simulink model "LCK"  (R2018b)
settings: Solver=FixedStepDiscrete  StartTime=0.0  StopTime=inf  FixedStep=0.01  RelTol=1e-3
PostLoadFcn:
  | if any(exist('dsrtsu_mdlpostloadfcn', 'file') ~= 0), dsrtsu_mdlpostloadfcn('Execute', bdroot); end
values from neighbouring files (symbols this model uses):
  C_DEG2RAD = 0.0175    [LCK_Macro.sldd]
  C_KPH2MPS = 0.2778    [LCK_Macro.sldd]
  C_NEARZERO = 0.0001    [LCK_Macro.sldd]
  C_ONE = 1.0    [LCK_Macro.sldd]
  C_RAD2DEG = 57.2958    [LCK_Macro.sldd]
  C_ZERO = 0.0    [LCK_Macro.sldd]
  k_accel_pedal_pos_per_speed_x : value not decoded    [LCK_LogicPara.sldd]
  k_accel_pedal_pos_per_speed_z : value not decoded    [LCK_LogicPara.sldd]
  k_brake_suprress_hold = 1000.0    [LCK_LogicPara.sldd]
  k_driver_appl_torque_filt = 50.0    [LCK_LogicPara.sldd]
  k_driver_suppression_hold_time = 3000.0    [LCK_LogicPara.sldd]
  k_hands_on_wheel_hold_msec = 500.0    [LCK_LogicPara.sldd]
  k_hands_on_wheel_torque_hi = 0.2    [LCK_LogicPara.sldd]
  k_hands_on_wheel_torque_lo = 0.15    [LCK_LogicPara.sldd]
  k_handsoff_delay_cycles = 50.0    [LCK_LogicPara.sldd]
  k_handsoff_torq_Lo_CR = 0.3    [LCK_LogicPara.sldd]
  k_handson_delay_cycles = 5.0    [LCK_LogicPara.sldd]
  k_HighAccel_suppress_hold = 3000.0    [LCK_LogicPara.sldd]
  k_HLR_suprress_hold = 3000.0    [LCK_LogicPara.sldd]
  k_hs_StrAng_CR_threshold_z : value not decoded    [LCK_LogicPara.sldd]
  k_LC_Exit_Switch = 0.0    [LCK_LogicPara.sldd]
  k_LCG_Configured = 1.0    [LCK_LogicPara.sldd]
  k_LCK_A0_Rdy2Act_UseConst = 0.0    [LCK_LogicPara.sldd]
  k_LCK_A0Fac_ActSta : value not decoded    [LCK_CtrlPara.sldd]
  k_LCK_A0Fac_DrvStm : value not decoded    [LCK_CtrlPara.sldd]
  k_LCK_A0Shift_LftCurv : value not decoded    [LCK_CtrlPara.sldd]
  k_LCK_A0Shift_RgtCurv : value not decoded    [LCK_CtrlPara.sldd]
  k_LCK_A0Shift_StraLan = 0.0    [LCK_CtrlPara.sldd]
  k_LCK_A0ShiftFac_Dy_LftCurv : value not decoded    [LCK_CtrlPara.sldd]
  k_LCK_A0ShiftFac_Dy_RgtCurv : value not decoded    [LCK_CtrlPara.sldd]
  k_LCK_A0ShiftFac_Vspd : value not decoded    [LCK_CtrlPara.sldd]
  k_LCK_accel_inhibit_thold = 35.0    [LCK_LogicPara.sldd]
  k_LCK_Active2Ready_Mask = 255.0    [LCK_LogicPara.sldd]
  k_LCK_CvatRateBks : value not decoded    [LCK_CtrlPara.sldd]
  k_LCK_CvatrBks : value not decoded    [LCK_CtrlPara.sldd]
  k_LCK_DFac_Dy : value not decoded    [LCK_CtrlPara.sldd]
  k_LCK_DFac_Dy_Curv : value not decoded    [LCK_CtrlPara.sldd]
  k_LCK_DFac_HaCurCen : value not decoded    [LCK_CtrlPara.sldd]
  k_LCK_DFac_HaCurSid : value not decoded    [LCK_CtrlPara.sldd]
  k_LCK_DFac_HadCurCen : value not decoded    [LCK_CtrlPara.sldd]
  k_LCK_DFac_HadCurSid : value not decoded    [LCK_CtrlPara.sldd]
  k_LCK_DFac_HadStrCen : value not decoded    [LCK_CtrlPara.sldd]
  k_LCK_DFac_HadStrSid : value not decoded    [LCK_CtrlPara.sldd]
  k_LCK_DFac_HaStrCen : value not decoded    [LCK_CtrlPara.sldd]
  k_LCK_DFac_HaStrSid : value not decoded    [LCK_CtrlPara.sldd]
  k_LCK_DFac_Rad : value not decoded    [LCK_CtrlPara.sldd]
  k_LCK_DFac_SA_CurCen : value not decoded    [LCK_CtrlPara.sldd]
  k_LCK_DFac_SA_CurSid : value not decoded    [LCK_CtrlPara.sldd]
  k_LCK_DFac_SA_StrCen : value not decoded    [LCK_CtrlPara.sldd]
  k_LCK_DFac_SA_StrSid : value not decoded    [LCK_CtrlPara.sldd]
  k_LCK_DFac_SS_CurCen : value not decoded    [LCK_CtrlPara.sldd]
  k_LCK_DFac_SS_CurSid : value not decoded    [LCK_CtrlPara.sldd]
  k_LCK_DFac_SS_StrCen : value not decoded    [LCK_CtrlPara.sldd]
  k_LCK_DFac_SS_StrSid : value not decoded    [LCK_CtrlPara.sldd]
  k_LCK_DFac_Vspd : value not decoded    [LCK_CtrlPara.sldd]
  k_LCK_DlyTm_DrvStim = 0.2    [LCK_CtrlPara.sldd]
  k_LCK_DTermMax = 2.0    [LCK_CtrlPara.sldd]
  k_LCK_DyBks_Curv : value not decoded    [LCK_CtrlPara.sldd]
  k_LCK_Enable_POOnly = 1.0    [LCK_LogicPara.sldd]
  k_LCK_Entry_DistBuffer = 0.1    [LCK_LogicPara.sldd]
  k_LCK_Fac_Vspd2RngThr_FalRec = 0.23    [LCK_CtrlPara.sldd]
  k_LCK_Ffw_CvatSwh = 0.0    [LCK_CtrlPara.sldd]
  k_LCK_Ffw_DyBks : value not decoded    [LCK_CtrlPara.sldd]
  k_LCK_Ffw_TimCon_CmdFlt = 0.0    [LCK_CtrlPara.sldd]
  k_LCK_FfwDeltaFac_Rad_Lft : value not decoded    [LCK_CtrlPara.sldd]
  k_LCK_FfwDeltaFac_Rad_Rgt : value not decoded    [LCK_CtrlPara.sldd]
  k_LCK_FfwDeltaFac_Vspd : value not decoded    [LCK_CtrlPara.sldd]
  k_LCK_FfwFac_CvatRate_Lft : value not decoded    [LCK_CtrlPara.sldd]
  k_LCK_FfwFac_CvatRate_Rgt : value not decoded    [LCK_CtrlPara.sldd]
  k_LCK_FfwFac_Dy : value not decoded    [LCK_CtrlPara.sldd]
  k_LCK_FfwFac_Rad_Lft : value not decoded    [LCK_CtrlPara.sldd]
  k_LCK_FfwFac_Rad_Rgt : value not decoded    [LCK_CtrlPara.sldd]
  k_LCK_FfwFac_Vspd : value not decoded    [LCK_CtrlPara.sldd]
  k_LCK_FfwTorq_Cvat : value not decoded    [LCK_CtrlPara.sldd]
  k_LCK_HAFac_ActSta : value not decoded    [LCK_CtrlPara.sldd]
  k_LCK_HAFac_DrvStm : value not decoded    [LCK_CtrlPara.sldd]
  k_LCK_HaloTime = 2000.0    [LCK_LogicPara.sldd]
  k_LCK_HaloTime_Switch = 0.0    [LCK_LogicPara.sldd]
  k_LCK_HARFac_ActSta : value not decoded    [LCK_CtrlPara.sldd]
  k_LCK_HARFac_DrvStm : value not decoded    [LCK_CtrlPara.sldd]
  k_LCK_Hed_DyBks : value not decoded    [LCK_CtrlPara.sldd]
  k_LCK_HedAngDiffX : value not decoded    [LCK_CtrlPara.sldd]
  k_LCK_HedAngRateDiffX : value not decoded    [LCK_CtrlPara.sldd]
  k_LCK_HndsOnWhel_DlyTm_Idl2Rdy = 0.0    [LCK_LogicPara.sldd]
  k_LCK_host_veh_width = 1.86    [LCK_LogicPara.sldd]
  k_LCK_Idle2Ready_Mask = 239.0    [LCK_LogicPara.sldd]
  k_LCK_Junc_SusTime = 1.0    [LCK_LogicPara.sldd]
  k_LCK_KpKdDecSlopeLmt = 10.0    [LCK_CtrlPara.sldd]
  k_LCK_KpKdIncSlopeLmt = 5.0    [LCK_CtrlPara.sldd]
  k_LCK_Lat_Ctrl_DFac_Lft = 1.0    [LCK_CtrlPara.sldd]
  k_LCK_Lat_Ctrl_DFac_Rgt = 1.05    [LCK_CtrlPara.sldd]
  k_LCK_Lat_Ctrl_Kd = 0.8    [LCK_CtrlPara.sldd]
  k_LCK_Lat_Ctrl_Ki = 0.5    [LCK_CtrlPara.sldd]
  k_LCK_Lat_Ctrl_Kp = 0.7    [LCK_CtrlPara.sldd]
  k_LCK_Lat_Ctrl_Kp_NearGain = 0.7    [LCK_CtrlPara.sldd]
  k_LCK_Lat_Ctrl_PFac_Lft = 1.0    [LCK_CtrlPara.sldd]
  k_LCK_Lat_Ctrl_PFac_Rgt = 1.05    [LCK_CtrlPara.sldd]
  k_LCK_Lat_Ctrl_TimCon_CmdFlt = 5.0    [LCK_CtrlPara.sldd]
  k_LCK_Lat_DFac_Rad : value not decoded    [LCK_CtrlPara.sldd]
  k_LCK_Lat_DFac_SS_Cur : value not decoded    [LCK_CtrlPara.sldd]
  k_LCK_Lat_DFac_SS_Str : value not decoded    [LCK_CtrlPara.sldd]
  k_LCK_Lat_DFac_Vspd : value not decoded    [LCK_CtrlPara.sldd]
  k_LCK_Lat_DyBks : value not decoded    [LCK_CtrlPara.sldd]
  k_LCK_Lat_IFac_Rad : value not decoded    [LCK_CtrlPara.sldd]
  k_LCK_Lat_IFac_Vspd : value not decoded    [LCK_CtrlPara.sldd]
  k_LCK_Lat_ILmtFac_Dy_CurvLan : value not decoded    [LCK_CtrlPara.sldd]
  k_LCK_Lat_ILmtFac_Dy_StraLan : value not decoded    [LCK_CtrlPara.sldd]
  k_LCK_Lat_ILmtFac_Rad : value not decoded    [LCK_CtrlPara.sldd]
  k_LCK_Lat_ILmtFac_Rad_NearGain = 1.0    [LCK_CtrlPara.sldd]
  k_LCK_Lat_ILmtFac_Vspd_CurvLan : value not decoded    [LCK_CtrlPara.sldd]
  k_LCK_Lat_ILmtFac_Vspd_StraLan : value not decoded    [LCK_CtrlPara.sldd]
  k_LCK_Lat_ITermLmt_Dy = 1.0    [LCK_CtrlPara.sldd]
  k_LCK_Lat_KpKdDecSlopeLmt = 10.0    [LCK_CtrlPara.sldd]
  k_LCK_Lat_KpKdIncSlopeLmt = 10.0    [LCK_CtrlPara.sldd]
  k_LCK_Lat_PFac_Dy_InnLftCur : value not decoded    [LCK_CtrlPara.sldd]
  k_LCK_Lat_PFac_Dy_InnRgtCur : value not decoded    [LCK_CtrlPara.sldd]
  k_LCK_Lat_PFac_Dy_OutLftCur : value not decoded    [LCK_CtrlPara.sldd]
  k_LCK_Lat_PFac_Dy_OutRgtCur : value not decoded    [LCK_CtrlPara.sldd]
  k_LCK_Lat_PFac_Dy_Str : value not decoded    [LCK_CtrlPara.sldd]
  k_LCK_Lat_PFac_Rad : value not decoded    [LCK_CtrlPara.sldd]
  ... (+153 more)
undefined symbols (not defined in the file or in its folder): k_LCK_CurvBks, K_LCK_SPA0A1A2_LMRngCmp_y
libraries: LateralControl_fcns_lib x59, simulink x24
(part 30 of 47)

== system LCK/Lateral_Control_Module/LCK_State_Ctrl/LCK_Mode_Transition/Determination_of_Junction ==
  SP_max_range : Inport
  VIS_LANE_LEFT_INDIVID_RANGE : Inport  Port=2
  VIS_LANE_RIGHT_INDIVID_RANGE : Inport  Port=3
  SP_type : Inport  Port=4
  Constant14 : Constant  Tag={'output',{'name','$P','class','EXTERN_MACRO','type','UInt8'},'date',737531.64011871524}  Description=_GACA26P4.LCK.000_9_  Value=TJA_SP_TYPE_BLMONLY
  Constant17 : Constant  Tag={'output',{'name','$P','class','EXTERN_MACRO','type','UInt8'},'date',737531.6327261111}  Description=_GACA26P4.LCK.000_10_  Value=TJA_SP_TYPE_BLMONLY
  Data Type Conversion88 : DataTypeConversion  Description=_GACA26P4.LCK.000_13_
  Data Type Conversion89 : DataTypeConversion  Description=_GACA26P4.LCK.000_14_
  Delay_Trig : LateralControl_fcns_lib/Delay_Trig  SystemSampleTime=-1
  Logical Operator155 : Logic  Tag={'date',737531.60590739583}  Description=_GACA26P4.LCK.000_31_  Operator=NOT  AllPortsSameDT=off  OutDataTypeStr=boolean
  Logical Operator157 : Logic  Tag={'date',737531.60590834497}  Description=_GACA26P4.LCK.000_32_  Inputs=3  AllPortsSameDT=off  OutDataTypeStr=boolean
  MinMax3 : MinMax  Tag={'output',{'type','Float32'},'date',737531.79517509264}  Description=_GACA26P4.LCK.000_35_  Inputs=2  OutDataTypeStr=single
  Relational Operator204 : RelationalOperator  Tag={'date',737531.60601302085}  Description=_GACA26P4.LCK.000_37_  Operator===  OutDataTypeStr=boolean  RndMeth=Nearest
  Relational Operator205 : RelationalOperator  Tag={'date',737531.60601353005}  Description=_GACA26P4.LCK.000_38_  Operator=<  OutDataTypeStr=boolean  RndMeth=Nearest
  Relational Operator207 : RelationalOperator  Tag={'date',737531.60601446754}  Description=_GACA26P4.LCK.000_39_  Operator===  OutDataTypeStr=boolean  RndMeth=Nearest
  Relational Operator208 : RelationalOperator  Tag={'date',737531.60601498839}  Description=_GACA26P4.LCK.000_40_  Operator=<  OutDataTypeStr=boolean  RndMeth=Nearest
  Relational Operator209 : RelationalOperator  Tag={'date',737531.60601548606}  Description=_GACA26P4.LCK.000_41_  Operator===  OutDataTypeStr=boolean  RndMeth=Nearest
  Signal_Sustain_With_Clear : LateralControl_fcns_lib/Signal_Sustain_With_Clear  Description=_GWMAB30P4.Latctrl.000_162_  SystemSampleTime=-1
  Switch67 : Switch  Tag={'output',{'type','Float32'},'threshold',{'type','Int32'},'date',737531.80936515052}  Description=_GACA26P4.LCK.000_47_  Threshold=0.5
  Switch69 : Switch  Tag={'output',{'type','Float32'},'threshold',{'type','Int32'},'date',737531.80957618053}  Description=_GACA26P4.LCK.000_49_  Threshold=0.5
  Unit Delay11 : UnitDelay  Tag={'output',{'inheritscaling',1},'state',{'type','Int32'},'date',737531.81173646986}  Description=_GACA26P4.LCK.000_54_  SampleTime=-1
  Unit Delay6 : UnitDelay  Tag={'output',{'inheritscaling',1},'state',{'type','Int32'},'date',737531.80972199072}  Description=_GACA26P4.LCK.000_55_  SampleTime=-1
  Unit Delay7 : UnitDelay  Tag={'output',{'inheritscaling',1},'state',{'type','Int32'},'date',737531.80965883099}  Description=_GACA26P4.LCK.000_56_  SampleTime=-1
  k_LCK_Junc_SusTime : Constant  Tag={'output',{'name','$P','class','EXTERN_CAL','type','Float32'},'date',737531.6374285185}  Description=_GACA26P4.LCK.000_59_  Value=k_LCK_Junc_SusTime
  k_LCK_MinJunction_Range : Constant  Tag={'output',{'name','$P','class','EXTERN_CAL','type','Float32'},'date',737531.63752556709}  Description=_GACA26P4.LCK.000_60_  Value=k_LCK_MinJunction_Range
  k_LCK_Range_Drop_MinDur : Constant  Tag={'output',{'name','$P','class','EXTERN_CAL','type','Float32'},'date',737531.63768747682}  Description=_GACA26P4.LCK.000_62_  Value=k_LCK_Range_Drop_MinDur
  k_LCK_UseSP_MaxRange : Constant  Tag={'output',{'name','$P','class','EXTERN_CAL','type','Bool'},'date',737531.64552409726}  Description=_GACA26P4.LCK.000_71_  Value=k_LCK_UseSP_MaxRange  VectorParams1D=off
  Junction : Outport
  wires:
  Relational Operator208/1 -> Logical Operator157/2
  Unit Delay6/1 -> Switch69/1
  Switch67/1 -> [LM_Range], Unit Delay7/1, Relational Operator209/1, Unit Delay11/1
  Switch69/1 -> Relational Operator205/2, Unit Delay6/1
  Relational Operator207/1 -> Logical Operator155/1
  Constant17/1 -> Relational Operator207/1
  [LM_Range] -> Relational Operator208/1
  Relational Operator205/1 -> Data Type Conversion89/1
  k_LCK_MinJunction_Range/1 -> Relational Operator208/2
  MinMax3/1 -> Switch67/3
  Logical Operator155/1 -> Data Type Conversion88/1
  k_LCK_Junc_SusTime/1 -> Signal_Sustain_With_Clear/2
  Delay_Trig/1 -> Signal_Sustain_With_Clear/1
  Constant14/1 -> Relational Operator204/1
  VIS_LANE_LEFT_INDIVID_RANGE/1 -> MinMax3/1
  Unit Delay11/1 -> Relational Operator209/2
  Signal_Sustain_With_Clear/1 -> Logical Operator157/3
  Logical Operator157/1 -> Junction/1
  Relational Operator204/1 -> Logical Operator157/1
  Data Type Conversion88/1 -> Signal_Sustain_With_Clear/3
  [SP_type] -> Relational Operator204/2
  Unit Delay7/1 -> Switch69/3
  [LM_Range] -> Relational Operator205/1
  Relational Operator209/1 -> Switch69/2
  k_LCK_UseSP_MaxRange/1 -> Switch67/2
  k_LCK_Range_Drop_MinDur/1 -> Delay_Trig/2
  Data Type Conversion89/1 -> Delay_Trig/1
  SP_type/1 -> [SP_type], Relational Operator207/2
  SP_max_range/1 -> Switch67/1
  VIS_LANE_RIGHT_INDIVID_RANGE/1 -> MinMax3/2

== system LCK/Lateral_Control_Module/LCK_State_Ctrl/LCK_Mode_Transition/Determination_of_Lat_Ctrl_Req ==
  LCK_Switch : Inport
  TJA_LatCtrl_Rq_Input : Inport  Port=2
  veh_speed_kph : Inport  Port=3
  Constant1 : Constant  Value=k_LCK_TJALCK_SWSpeed
  Constant20 : Constant  Tag={'output',{'type','Int32'},'date',737184.60397293977}  Description=_GWMAB30P2.LCK.000_1071_
  LCK_TJA_LatRq_Manager : Stateflow chart  TreatAsAtomicUnit=on
  Switch6 : Switch  Tag={'output',{'inheritscaling',1},'threshold',{'type','Int32','scalar',1},'date',737243.50339983799}  Description=_GWMAB30P2.LCK.000_1196_  Threshold=0.5
  k_LCK_VisionOnly : Constant  Tag={'output',{'name','$P','class','EXTERN_CAL','type','Bool'},'date',737246.86429052078}  Description=_GWMAB30P2.LCK.000_1268_  Value=k_LCK_VisionOnly
  LCKON_TJAOFF : Outport
  TJA_LatCtrl_Rq : Outport  Port=2
  wires:
  veh_speed_kph/1 -> LCK_TJA_LatRq_Manager/3(VehicleSpd)
  Constant20/1 -> Switch6/1
  k_LCK_VisionOnly/1 -> Switch6/2
  Switch6/1 -> TJA_LatCtrl_Rq/1
  Constant1/1 -> LCK_TJA_LatRq_Manager/4(k_LCK_TJALCK_SWSpeed)
  LCK_TJA_LatRq_Manager/2(LatRq) -> Switch6/3
  TJA_LatCtrl_Rq_Input/1 -> LCK_TJA_LatRq_Manager/1(TJA_LatCtrl_Rq)
  LCK_TJA_LatRq_Manager/1(LCKON_TJAOFF) -> LCKON_TJAOFF/1
  LCK_Switch/1 -> LCK_TJA_LatRq_Manager/2(LCK_Switch)

== system LCK/Lateral_Control_Module/LCK_State_Ctrl/LCK_Mode_Transition/Determination_of_OFF2IDLE ==
  TJA_Switch : Inport
  LCK_Switch : Inport  Port=2
  Logical Operator : Logic  Tag={'date',737184.60397559032}  Description=_GWMAB30P2.LCK.000_1090_  Operator=OR  AllPortsSameDT=off  OutDataTypeStr=boolean
  OFF2IDLE : Outport
  wires:
  TJA_Switch/1 -> Logical Operator/1
  LCK_Switch/1 -> Logical Operator/2
  Logical Operator/1 -> OFF2IDLE/1

== system LCK/Lateral_Control_Module/LCK_State_Ctrl/LCK_Mode_Transition/Determination_of_OFF2READY ==
  TJA_Switch : Inport
  LCK_Switch : Inport  Port=2
  IDLE2READY : Inport  Port=3
  Logical Operator48 : Logic  Tag={'date',737237.63746775466}  Description=_GWMAB30P3.LCK.000_66_  Operator=OR  AllPortsSameDT=off  OutDataTypeStr=boolean
  Logical Operator49 : Logic  Tag={'date',737237.63746789354}  Description=_GWMAB30P3.LCK.000_67_  Inputs=3  AllPortsSameDT=off  OutDataTypeStr=boolean
  Relational_Operator6 : RelationalOperator  Tag={'date',737237.63747481478}  Description=_GWMAB30P3.LCK.000_109_  Operator===  OutDataTypeStr=boolean  RndMeth=Nearest
  ZERO7 : Constant  Tag={'output',{'type','Int32'},'date',737296.79743047454}  Description=_GWMAB30P3.LCK.000_124_  Value=0  SampleTime=-1
  OFF2READY : Outport
  wires:
  IDLE2READY/1 -> Logical Operator49/2
  Logical Operator48/1 -> Logical Operator49/1
  TJA_Switch/1 -> Logical Operator48/1
  ZERO7/1 -> Relational_Operator6/2
  [LCK_VisionOnly] -> Relational_Operator6/1
  Logical Operator49/1 -> OFF2READY/1
  LCK_Switch/1 -> Logical Operator48/2
  Relational_Operator6/1 -> Logical Operator49/3
